simulink model "JayaMPPT"  (R2020a)
settings: Solver=VariableStepAuto  StartTime=0.0  StopTime=0.3  RelTol=1e-4
libraries: powerlib x13, re_lib x3, powerlib_meascontrol x1, simulink x1
settings Model: Creator=Admin  LastModifiedBy=Admin
settings SolverCC: ZeroCrossAlgorithm=Adaptive
settings DataIOCC: ReturnWorkspaceOutputsName=Jaya
settings DebuggingCC: IgnoredZcDiagnostic=none

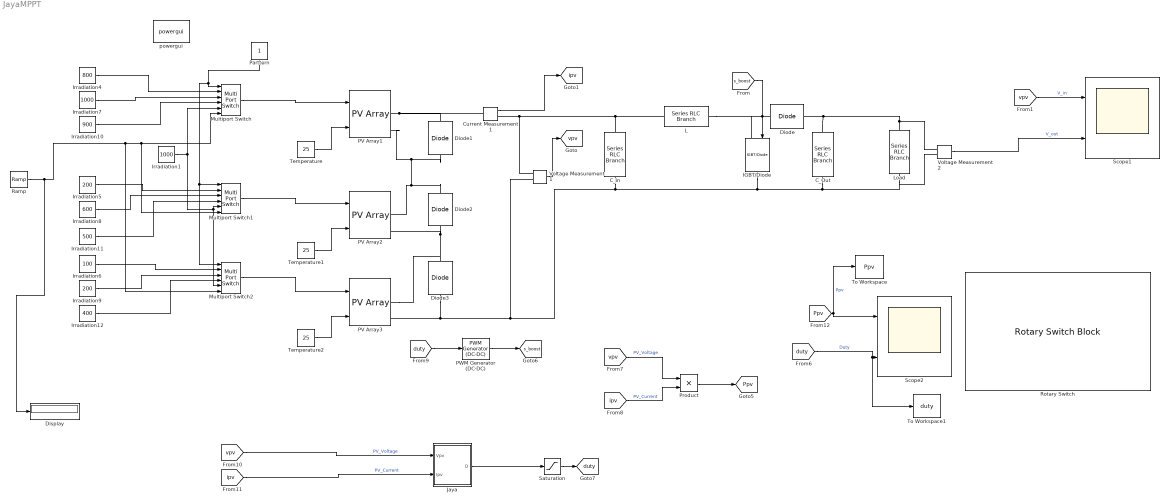
== system JayaMPPT ==
  C_Out : powerlib/Elements/Series RLC Branch  LConnTagsString=__new0  RConnTagsString=__new0  BranchType=C  Resistance=1e-4  Inductance=1e-3  SetiL0=off  InitialCurrent=0  Capacitance=7.76393e-6  Setx0=off  InitialVoltage=0  Measurements=None
  C_in : powerlib/Elements/Series RLC Branch  LConnTagsString=__new0  RConnTagsString=__new0  BranchType=C  Resistance=1e-4  Inductance=1e-3  SetiL0=off  InitialCurrent=0  Capacitance=1.76631e-4  Setx0=off  InitialVoltage=0  Measurements=None
  Current Measurement1 : powerlib/Measurements/Current Measurement  PhasorSimulation=off  OutputType=Complex  PSBequivalent=0
  Diode : powerlib/Power Electronics/Diode  Ron=0.001  Lon=0  Vf=0.8  IC=0  UseSnubber=0  Rs=500  Cs=250e-9  Measurements=off
  Diode1 : powerlib/Power Electronics/Diode  Ron=0.001  Lon=0  Vf=0.6  IC=0  UseSnubber=0  Rs=500  Cs=250e-9  Measurements=off
  Diode2 : powerlib/Power Electronics/Diode  Ron=0.001  Lon=0  Vf=0.6  IC=0  UseSnubber=0  Rs=500  Cs=250e-9  Measurements=off
  Diode3 : powerlib/Power Electronics/Diode  Ron=0.001  Lon=0  Vf=0.6  IC=0  UseSnubber=0  Rs=500  Cs=250e-9  Measurements=off
  Display : Display
  IGBT/Diode : powerlib/Power Electronics/IGBT//Diode  Ron=1  Rs=1e5  Cs=inf  Measurements=off
  Irradiation1 : Constant  Value=1000
  Irradiation10 : Constant  Value=900
  Irradiation11 : Constant  Value=500
  Irradiation12 : Constant  Value=400
  Irradiation4 : Constant  Value=800
  Irradiation5 : Constant  Value=200
  Irradiation6 : Constant  Value=100
  Irradiation7 : Constant  Value=1000
  Irradiation8 : Constant  Value=600
  Irradiation9 : Constant  Value=200
  Jaya : MATLAB Function  TreatAsAtomicUnit=on
  L : powerlib/Elements/Series RLC Branch  LConnTagsString=__new0  RConnTagsString=__new0  BranchType=L  Resistance=0.1  Inductance=0.0000213337  SetiL0=off  InitialCurrent=0  Capacitance=100e-6  Setx0=off  InitialVoltage=0  Measurements=None
  Load : powerlib/Elements/Series RLC Branch  LConnTagsString=__new0  RConnTagsString=__new0  BranchType=R  Resistance=30  Inductance=1e-3  SetiL0=off  InitialCurrent=0  Capacitance=3300e-6  Setx0=off  InitialVoltage=0  Measurements=None
  Multiport Switch : MultiPortSwitch  Inputs=5
  Multiport Switch1 : MultiPortSwitch  Inputs=5
  Multiport Switch2 : MultiPortSwitch  Inputs=5
  PV Array1 : re_lib/Solar/PV Array  Npar=1  Nser=1  PlotType=array @ 25 deg.C & specified irradiances  S_vec=[ 1000 800 600 400 200]  Temp_C_vec="[ 45 25  ]"  ModuleName=User-defined  PlotWhenSelected=off  Pm=260.224  Ncell=60  Voc=37.5  Isc=9.12  Vm=30.4  Im=8.56  beta_Voc_pc=-0.31  alpha_Isc_pc=0.053  beta_Voc=-0.11625  alpha_Isc=0.0048336  IL=9.1977  I0=4.7278e-11  nI=0.93687  Rsh=146.6161  Rs=0.32023  RobustModel=off  RobustCellTemperature=25  BAL=on  Tc=1e-5  Tfilter=5e-5
  PV Array2 : re_lib/Solar/PV Array  Npar=1  Nser=1  PlotType=array @ 25 deg.C & specified irradiances  S_vec=[ 1000 800 600 400 200]  Temp_C_vec="[ 45 25  ]"  ModuleName=User-defined  PlotWhenSelected=off  Pm=260.224  Ncell=60  Voc=37.5  Isc=9.12  Vm=30.4  Im=8.56  beta_Voc_pc=-0.31  alpha_Isc_pc=0.053  beta_Voc=-0.11625  alpha_Isc=0.0048336  IL=9.1977  I0=4.7278e-11  nI=0.93687  Rsh=146.6161  Rs=0.32023  RobustModel=off  RobustCellTemperature=25  BAL=on  Tc=1e-5  Tfilter=5e-5
  PV Array3 : re_lib/Solar/PV Array  Npar=1  Nser=1  PlotType=array @ 25 deg.C & specified irradiances  S_vec=[ 1000 800 600 400 200]  Temp_C_vec="[ 45 25  ]"  ModuleName=User-defined  PlotWhenSelected=off  Pm=260.224  Ncell=60  Voc=37.5  Isc=9.12  Vm=30.4  Im=8.56  beta_Voc_pc=-0.31  alpha_Isc_pc=0.053  beta_Voc=-0.11625  alpha_Isc=0.0048336  IL=9.1977  I0=4.7278e-11  nI=0.93687  Rsh=146.6161  Rs=0.32023  RobustModel=off  RobustCellTemperature=25  BAL=on  Tc=1e-5  Tfilter=5e-5
  PWM Generator (DC-DC) : powerlib_meascontrol/Pulse & Signal Generators/PWM Generator (DC-DC)  Fsw=50000  Ts=0
  "Parttern " : Constant
  Product : Product
  Ramp : simulink/Sources/Ramp  slope=-2000  start=0  InitialOutput=1000  VectorParams1D=off
  Rotary Switch : RotarySwitchBlock
      settings: Values={{'1', '2', '3', 'STC', 'Change IR'}, [1 2 3 4 5]}
  Saturation : Saturate  UpperLimit=1  LowerLimit=0
  Scope1 : Scope  NumInputPorts=2
  Scope2 : Scope  NumInputPorts=2
  Temperature : Constant  Value=25
  Temperature1 : Constant  Value=25
  Temperature2 : Constant  Value=25
  To Workspace : ToWorkspace  VariableName=Ppv  SaveFormat=Timeseries  SampleTime=-1
      settings: Save2DSignal=2-D array (concatenate along first dimension)
  To Workspace1 : ToWorkspace  VariableName=duty  SaveFormat=Timeseries  SampleTime=-1
      settings: Save2DSignal=2-D array (concatenate along first dimension)
  Voltage Measurement1 : powerlib/Measurements/Voltage Measurement  PhasorSimulation=off  OutputType=Complex  PSBequivalent=0
  Voltage Measurement2 : powerlib/Measurements/Voltage Measurement  PhasorSimulation=off  OutputType=Complex  PSBequivalent=0
  powergui : powerlib/powergui  Priority=1  SimulationMode=Continuous  SampleTime=1e-06  frequency=60  Iterations=50  frequencyindice=0  Pbase=100e6  ErrMax=1e-4  UnitsV=kV  UnitsW=MW  buscounter=0  FunctionMessages=off  echomessages=off  EnableUseOfTLC=off  CurrentSourceSwitches=off  DisableSnubberDevices=off  DisableRonSwitches=off  DisableVfSwitches=off  DisplayEquations=off  AutomaticDiscreteSolvers=off  SolverType=Tustin/Backward Euler (TBE)  Interpol=off  ExternalGateDelay=off  methode=off  Ts=10  x0status=blocks  SPID=off  SwTol=0  HookPort=off  NonlinearTolerance=0  nMaxIteration=15  ContinueOnMaxIteration=off  RestoreLinks=warning  ResistiveCurrentMeasurement=off  Frange=[0:2:500]  Ylog=off  Xlog=on  ShowGrid=off  save=off  variable=ZData  structure=0  ZoomFFT=off  StartTime=0.0  cycles=1  DisplayStyle=1  fundamental=60  FreqAxis=off  MaxFrequency=1000  frequencyindicesteady=1  RmsSteady=1  display=off
  tag scope: Ppv=global, duty=global, ipv=global, s_boost=global, vpv=global
  wires:
  [vpv] -> Jaya/1(Vpv)  "PV_Voltage"
  Irradiation12/1 -> Multiport Switch2/4
  Irradiation5/1 -> Multiport Switch1/2
  Irradiation7/1 -> Multiport Switch/3
  Product/1 -> [Ppv]
  Irradiation6/1 -> Multiport Switch2/2
  [ipv] -> Product/2  "PV_Current"
  "Parttern "/1 -> Multiport Switch2/1, Multiport Switch1/1, Multiport Switch/1
  Temperature2/1 -> PV Array3/2
  Irradiation4/1 -> Multiport Switch/2
  Irradiation10/1 -> Multiport Switch/4
  [duty] -> PWM Generator (DC-DC)/1
  Irradiation8/1 -> Multiport Switch1/3
  [vpv] -> Product/1  "PV_Voltage"
  Irradiation9/1 -> Multiport Switch2/3
  [ipv] -> Jaya/2(Ipv)  "PV_Current"
  Multiport Switch2/1 -> PV Array3/1
  Saturation/1 -> [duty]
  Temperature/1 -> PV Array1/2
  Multiport Switch1/1 -> PV Array2/1
  Irradiation11/1 -> Multiport Switch1/4
  Voltage Measurement1/1 -> [vpv]
  PWM Generator (DC-DC)/1 -> [s_boost]
  Ramp/1 -> Display/1, Multiport Switch2/6, Multiport Switch/6, Multiport Switch1/6
  [Ppv] -> To Workspace/1, Scope2/1  "Ppv"
  Temperature1/1 -> PV Array2/2
  Current Measurement1/1 -> [ipv]
  Multiport Switch/1 -> PV Array1/1
  [s_boost] -> IGBT/Diode/1
  Irradiation1/1 -> Multiport Switch2/5, Multiport Switch1/5, Multiport Switch/5
  Jaya/1(D) -> Saturation/1
  [duty] -> To Workspace1/1, Scope2/2  "Duty"
  [vpv] -> Scope1/1  "V_in"
  Voltage Measurement2/1 -> Scope1/2  "V_out"
  connections:
  PV Array1/RConn2 -- Diode1/LConn1 -- PV Array2/RConn1 -- Diode2/RConn1
  PV Array1/RConn1 -- Diode1/RConn1 -- Current Measurement1/LConn1
  C_Out/RConn1 -- Voltage Measurement2/LConn2 -- Load/RConn1 -- IGBT/Diode/RConn1 -- C_in/RConn1 -- Diode3/LConn1 -- PV Array3/RConn2 -- Voltage Measurement1/LConn2
  C_in/LConn1 -- L/LConn1 -- Voltage Measurement1/LConn1 -- Current Measurement1/RConn1
  Diode2/LConn1 -- PV Array2/RConn2 -- PV Array3/RConn1 -- Diode3/RConn1
  C_Out/LConn1 -- Voltage Measurement2/LConn1 -- Load/LConn1 -- Diode/RConn1
  Diode/LConn1 -- IGBT/Diode/LConn1 -- L/RConn1

== matlab function JayaMPPT/Jaya ==
  settings: updateMethod=DISCRETE
  data: Vpv input; D output; Ipv input
function D = Jaya(Vpv, Ipv)
    coder.extrinsic('randi')
    
    persistent k p dc dcPrev Pbest Pprev dcurrent u ;
    P = Ipv * Vpv;
    if isempty(dc)
        k = 0;
        dc = zeros(3,1);

        dc(1)=randi( [5 330])/1000;
        dc(2)=randi( [330 660])/1000;
        dc(3)=randi( [660 995])/1000;
        
        dcPrev = dc;
        p = zeros(3,1);
        Pbest = Ipv * Vpv;
        Pprev = 0;
        dcurrent = 0.5;
        u=0;
    end
    
    D = dcurrent;
    
    if (P > Pbest)
        Pbest = P;        
    end
    if (k < 300)
        k=k+1;
        return;
    else
        k=0;
    end
    %{
    if abs(P - Pprev) < 1
       if abs(P - Pbest) > 15
          dc(1)=randi( [5 330])/1000;
          dc(2)=randi( [330 660])/1000;
          dc(3)=randi( [660 995])/1000;
          p = zeros(3,1);
          u= 0;
       end
    end
    %}
    if(u>=1 && u<=3)
        if(P>p(u))
            p(u)=P;
        else
            dc(u) = dcPrev(u);
        end
    end
    
    u=u+1;
    
    if (u > 4)
        u=1;
    end
    
    if (u == 4)
        [~,idx1]=max(p);
        dcBest = dc(idx1);
        [~,idx2]=min(p);
        dcWorst = dc(idx2);
        D = dcBest;
        dcPrev = dc;
        for j=1:3
            dc(j)= updateduty(dc(j),dcBest,dcWorst);
        end
    else
        D=dc(u);
        dcurrent = dc(u);
        Pprev = P;
    end
end
    
function dfinal=updateduty(d,d_best,d_worst)
    r1 = rand();
    r2 = rand();
    dfinal = d + r1*(d_best - abs(d)) - r2*(d_worst - abs(d));
    if dfinal > 1
        dfinal = 0.95;
    elseif dfinal <0
        dfinal = 0.05;
    end
end
